simulink model "bh_SL_test_algorithm_and_virtual_camera"  (R2017b)
settings: Solver=FixedStepDiscrete  StartTime=0.0  StopTime=33  RelTol=1e-3
PreLoadFcn:
  | bh_create_cv_neareset_BUS_OBJ_for_simulink()
  | fprintf('\n\n### just did a preload TASK !');
undefined symbols (not defined in the file or in its folder): gray
libraries: visiongeotforms x1, bh_cv_car_drc_library x1
settings Model: FPTRunName=Active  ExtModeAutoUpdateStatusClock=off  Creator=The MathWorks, Inc.  LastModifiedBy=bhorton
settings DataIOCC: LimitDataPoints=on  SaveFormat=Array  SaveOutput=off  SaveTime=off  SignalLoggingName=sigsOut
settings OptimizationCC: ExpressionDepthLimit=2147483647  InitFltsAndDblsToZero=on  LifeSpan=inf  BufferReusableBoundary=off
settings DebuggingCC: SaveWithParameterizedLinksMsg=none  UnderspecifiedInitializationDetection=Classic  MergeDetectMultiDrivingBlocksExec=none  CheckExecutionContextPreStartOutputMsg=on  CheckExecutionContextRuntimeOutputMsg=on  SignalResolutionControl=TryResolveAllWithWarning  MultiTaskDSMMsg=warning  MultiTaskCondExecSysMsg=none  ParameterPrecisionLossMsg=none  FcnCallInpInsideContextMsg=warning  BusObjectLabelMismatch=none  StateNameClashWarn=warning  StrictBusMsg=None  SFUnexpectedBacktrackingDiag=warning  SFNoUnconditionalDefaultTransitionDiag=warning  SFExecutionAtInitializationDiag=none
settings HardwareCC: ProdBitPerPointer=32  ProdBitPerSizeT=32  ProdBitPerPtrDiffT=32  ProdLargestAtomicFloat=None  ProdIntDivRoundTo=Undefined  ProdEndianess=Unspecified  ProdWordSize=32  ProdHWDeviceType=32-bit Generic  TargetBitPerPointer=64  TargetBitPerSizeT=64  TargetBitPerPtrDiffT=64  TargetLongLongMode=on  TargetIntDivRoundTo=Zero  TargetEndianess=LittleEndian  TargetWordSize=64  TargetHWDeviceType=Generic->MATLAB Host Computer  ProdEqTarget=off
settings ModelReferenceCC: PropagateSignalLabelsOutOfModel=off
settings CodeAppCC: StateflowObjectComments=on
settings GRTTargetCC: TargetFcnLib=ansi_tfl_tmw.mat  TargetLangStandard=C89/C90 (ANSI)  GeneratePreprocessorConditionals=Disable all  CombineOutputUpdateFcns=off  GRTInterface=on
settings ConfigComp: CovMetricSettings=dw  CovHtmlReporting=on  CovSaveCumulativeToWorkspaceVar=on  CovSaveSingleToWorkspaceVar=on  CovExternalEMLEnable=off

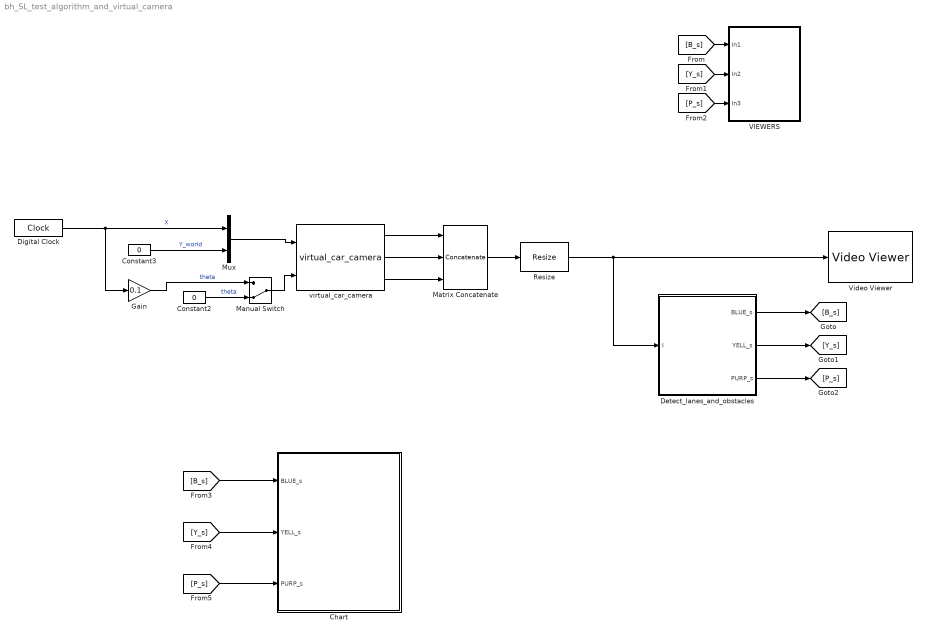
== system bh_SL_test_algorithm_and_virtual_camera ==
  Chart : Stateflow chart  TreatAsAtomicUnit=on
  Constant2 : Constant  Value=0
  Constant3 : Constant  Value=0
  Detect_lanes_and_obstacles : Subsystem
  Digital Clock : DigitalClock  SampleTime=0.1
  Gain : Gain  Gain=0.1
  Manual Switch : ManualSwitch  CurrentSetting=0
  Matrix Concatenate : Concatenate  NumInputs=3  Mode=Multidimensional array  ConcatenateDimension=3
  Mux : Mux  Inputs=2
  Resize : visiongeotforms/Resize  specify=Number of output rows and columns  rfactor=[180 240]  outCols=25  outRows=25  outRowsCols=[180 240]  interp_method=Bilinear  antialias=off  useROI=off  roiFlag=off  prodOutputMode=Binary point scaling  prodOutputWordLength=32  prodOutputFracLength=10  roundingMode=Nearest  overflowMode=on
      settings: SourceProductName=Computer Vision System Toolbox  SourceProductBaseCode=VP
  VIEWERS : Subsystem
  Video Viewer : VideoViewer  colormapValue=gray(256)  FigPos=[2034 1219 418 304]
  virtual_car_camera : bh_cv_car_drc_library/CAR_things/virtual_car_camera  W=320  H=240  Ts=0.1  init_cam_pos_wrt_W=[0,0]  height_of_cam=0.4  init_veh_THETA_wrt_W=0  horz_look_dist=11  cam_va=45
  wires:
  Matrix Concatenate/1 -> Resize/1
  Resize/1 -> Detect_lanes_and_obstacles/1(I), Video Viewer/1
  Mux/1 -> virtual_car_camera/1
  Gain/1 -> Manual Switch/1  "theta"
  virtual_car_camera/3 -> Matrix Concatenate/3
  virtual_car_camera/1 -> Matrix Concatenate/1
  Constant2/1 -> Manual Switch/2  "theta"
  virtual_car_camera/2 -> Matrix Concatenate/2
  Digital Clock/1 -> Gain/1, Mux/1  "X"
  Constant3/1 -> Mux/2  "Y_world"
  Manual Switch/1 -> virtual_car_camera/2
  Detect_lanes_and_obstacles/1(BLUE_s) -> [B_s]
  Detect_lanes_and_obstacles/2(YELL_s) -> [Y_s]
  Detect_lanes_and_obstacles/3(PURP_s) -> [P_s]
  [P_s] -> VIEWERS/3(In3)
  [Y_s] -> VIEWERS/2(In2)
  [B_s] -> VIEWERS/1(In1)
  [P_s] -> Chart/3(PURP_s)
  [Y_s] -> Chart/2(YELL_s)
  [B_s] -> Chart/1(BLUE_s)

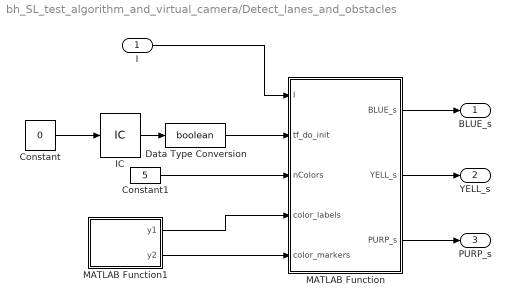
== system bh_SL_test_algorithm_and_virtual_camera/Detect_lanes_and_obstacles ==
  I : Inport
  Constant : Constant  Value=0  OutDataTypeStr=boolean
  Constant1 : Constant  Value=5  OutDataTypeStr=double
  Data Type Conversion : DataTypeConversion  OutDataTypeStr=boolean
  IC : InitialCondition
  MATLAB Function : MATLAB Function  TreatAsAtomicUnit=on
  MATLAB Function1 : MATLAB Function  TreatAsAtomicUnit=on
  BLUE_s : Outport
  YELL_s : Outport  Port=2
  PURP_s : Outport  Port=3
  wires:
  Constant/1 -> IC/1
  Data Type Conversion/1 -> MATLAB Function/2(tf_do_init)
  IC/1 -> Data Type Conversion/1
  Constant1/1 -> MATLAB Function/3(nColors)
  MATLAB Function1/1(y1) -> MATLAB Function/4(color_labels)
  MATLAB Function1/2(y2) -> MATLAB Function/5(color_markers)
  I/1 -> MATLAB Function/1(I)
  MATLAB Function/3(PURP_s) -> PURP_s/1
  MATLAB Function/2(YELL_s) -> YELL_s/1
  MATLAB Function/1(BLUE_s) -> BLUE_s/1

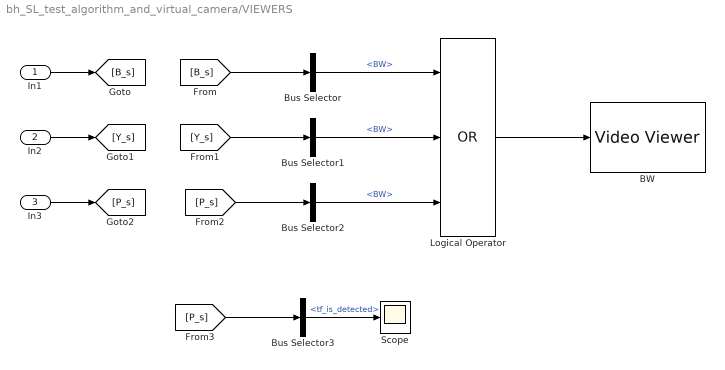
== system bh_SL_test_algorithm_and_virtual_camera/VIEWERS ==
  In1 : Inport
  In2 : Inport  Port=2
  In3 : Inport  Port=3
  BW : VideoViewer  colormapValue=gray(256)  FigPos=[2041 741 418 304]
  Bus Selector : BusSelector  OutputSignals=BW
  Bus Selector1 : BusSelector  OutputSignals=BW
  Bus Selector2 : BusSelector  OutputSignals=BW
  Bus Selector3 : BusSelector  OutputSignals=tf_is_detected
  Logical Operator : Logic  Operator=OR  Inputs=3  AllPortsSameDT=off  OutDataTypeStr=boolean
  Scope : Scope
  wires:
  [P_s] -> Bus Selector2/1
  [B_s] -> Bus Selector/1
  Logical Operator/1 -> BW/1
  [Y_s] -> Bus Selector1/1
  Bus Selector/1 -> Logical Operator/1  "<BW>"
  Bus Selector1/1 -> Logical Operator/2  "<BW>"
  Bus Selector2/1 -> Logical Operator/3  "<BW>"
  In3/1 -> [P_s]
  In2/1 -> [Y_s]
  In1/1 -> [B_s]
  [P_s] -> Bus Selector3/1
  Bus Selector3/1 -> Scope/1  "<tf_is_detected>"

== matlab function bh_SL_test_algorithm_and_virtual_camera/Detect_lanes_and_obstacles/MATLAB Function1 ==
  data: y1 output; y2 output
function [y1, y2] = fcn()

y1 = [0,1,2,3,4];

y2 = [ ...
       -7.8436  -30.0394;
      -10.2908   36.4110;
       42.5297   -8.7231;
        2.1904    1.6907;
        4.0686    3.2113;
        ];
    
end

== matlab function bh_SL_test_algorithm_and_virtual_camera/Detect_lanes_and_obstacles/MATLAB Function ==
  data: I input; BLUE_s output Bus: lane_info_BUS; tf_do_init input; YELL_s output Bus: lane_info_BUS; PURP_s output Bus: box_info_BUS; nColors input; color_labels input; color_markers input
function [BLUE_s, YELL_s, PURP_s] = fcn(I, tf_do_init, ...
                                        nColors, color_labels, color_markers)

coder.extrinsic('bh_my_ALGORITHM_for_codegen')

marker_s.nColors       = nColors;
marker_s.color_labels  = color_labels;
marker_s.color_markers = color_markers;

[BLUE_s, YELL_s, PURP_s] = bh_my_ALGORITHM_for_codegen(I, tf_do_init, marker_s);

end

== stateflow chart bh_SL_test_algorithm_and_virtual_camera/Chart ==
  state DETECTION_SUMMARY
    state OUTER [parallel]
      settings: executionOrder=1
      state NOT_Detected
      state Detected
      (default) -> (junction 15)
      (junction 15) -> DETECTION_SUMMARY.OUTER.NOT_Detected [order 1] : [~BLUE_s.tf_is_detected]
      (junction 15) -> DETECTION_SUMMARY.OUTER.Detected [order 2] : [BLUE_s.tf_is_detected]
      DETECTION_SUMMARY.OUTER.NOT_Detected -> DETECTION_SUMMARY.OUTER.Detected : [BLUE_s.tf_is_detected]
      DETECTION_SUMMARY.OUTER.Detected -> DETECTION_SUMMARY.OUTER.NOT_Detected : [~BLUE_s.tf_is_detected]
    state INNER [parallel]
      settings: executionOrder=2
      state NOT_Detected
      state Detected
      (default) -> (junction 30)
      (junction 30) -> DETECTION_SUMMARY.INNER.NOT_Detected [order 1] : [~YELL_s.tf_is_detected]
      (junction 30) -> DETECTION_SUMMARY.INNER.Detected [order 2] : [YELL_s.tf_is_detected]
      DETECTION_SUMMARY.INNER.NOT_Detected -> DETECTION_SUMMARY.INNER.Detected : [YELL_s.tf_is_detected]
      DETECTION_SUMMARY.INNER.Detected -> DETECTION_SUMMARY.INNER.NOT_Detected : [~YELL_s.tf_is_detected]
    state PURPLE [parallel]
      settings: executionOrder=3
      state NOT_Detected
      state Detected
      (default) -> (junction 41)
      (junction 41) -> DETECTION_SUMMARY.PURPLE.NOT_Detected [order 1] : [~PURP_s.tf_is_detected]
      (junction 41) -> DETECTION_SUMMARY.PURPLE.Detected [order 2] : [PURP_s.tf_is_detected]
      DETECTION_SUMMARY.PURPLE.NOT_Detected -> DETECTION_SUMMARY.PURPLE.Detected : [PURP_s.tf_is_detected]
      DETECTION_SUMMARY.PURPLE.Detected -> DETECTION_SUMMARY.PURPLE.NOT_Detected : [~PURP_s.tf_is_detected]
    state ? [parallel] [commented out]
  (default) -> DETECTION_SUMMARY
  data: BLUE_s input Bus: lane_info_BUS; YELL_s input Bus: lane_info_BUS; PURP_s input Bus: box_info_BUS
